simulink model "screening_workflow"  (Simulink 10.0)
values from neighbouring files (symbols this model uses):
  ai_daily_capacity = floor((24 * 3600) / max(0.5, ai_inference_time_sec))    [run_simulation.m]
  bandwidth_daily_capacity = floor((10 * 3600) / max(1.0, sec_per_upload))    [run_simulation.m]
  images_per_day_per_camera = 40    [build_telemedicine_model.m]    (also in run_simulation.m)
  num_cameras = 5    [build_telemedicine_model.m]    (also in run_simulation.m)
  reviewer_daily_capacity = floor(num_reviewers * (reviewer_daily_sec / max(5, avg_review_time_sec)))    [run_simulation.m]
settings Model: OverrideTechnique=None  ModelVersion=1.42

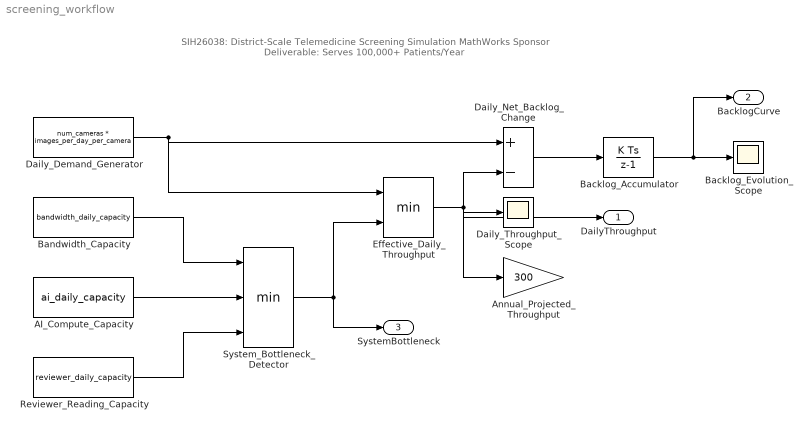
== system screening_workflow ==
  note: SIH26038: District-Scale Telemedicine Screening Simulation
      | MathWorks Sponsor Deliverable: Serves 100,000+ Patients/Year
  Daily_Demand_Generator : Constant  Value=num_cameras * images_per_day_per_camera
  Bandwidth_Capacity : Constant  Value=bandwidth_daily_capacity
  AI_Compute_Capacity : Constant  Value=ai_daily_capacity
  Reviewer_Reading_Capacity : Constant  Value=reviewer_daily_capacity
  System_Bottleneck_Detector : MinMax  Function=min  Inputs=3  InputSameDT=off
  Effective_Daily_Throughput : MinMax  Function=min  Inputs=2  InputSameDT=off
  Daily_Net_Backlog_Change : Sum  Inputs=+-
  Backlog_Accumulator : DiscreteIntegrator  IntegratorMethod=Integration: Forward Euler  ExternalReset=none  InitialConditionSource=internal  InitialCondition=0  LimitOutput=on  UpperSaturationLimit=100000  LowerSaturationLimit=0  SampleTime=1
  Annual_Projected_Throughput : Gain  Gain=300
  Backlog_Evolution_Scope : Scope
      settings: ShowLegends=on  TimeRange=365  YMin=0  YMax=5000  SaveName=ScopeData
  Daily_Throughput_Scope : Scope
      settings: ShowLegends=on  TimeRange=365  SaveName=ScopeDataThroughput
  DailyThroughput : Outport
  BacklogCurve : Outport  Port=2
  SystemBottleneck : Outport  Port=3
  wires:
  Daily_Demand_Generator/1 -> Daily_Net_Backlog_Change/1, Effective_Daily_Throughput/1
  Bandwidth_Capacity/1 -> System_Bottleneck_Detector/1
  AI_Compute_Capacity/1 -> System_Bottleneck_Detector/2
  Reviewer_Reading_Capacity/1 -> System_Bottleneck_Detector/3
  System_Bottleneck_Detector/1 -> Effective_Daily_Throughput/2, SystemBottleneck/1
  Effective_Daily_Throughput/1 -> Daily_Net_Backlog_Change/2, Daily_Throughput_Scope/1, DailyThroughput/1, Annual_Projected_Throughput/1
  Daily_Net_Backlog_Change/1 -> Backlog_Accumulator/1
  Backlog_Accumulator/1 -> Backlog_Evolution_Scope/1, BacklogCurve/1
